simulink model "ModeloLineal_ex1"  (R2025b)
settings: Solver=VariableStepAuto  StartTime=0.0  StopTime=10.0  RelTol=1e-3
undefined symbols (not defined in the file): A, Gain, Gain2
settings Model: Creator=NMB  LastModifiedBy=NMB

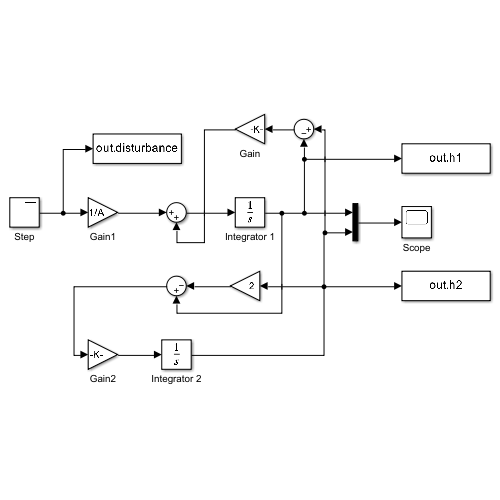
[thumbnail: Simulink's stored preview of the top-level diagram]
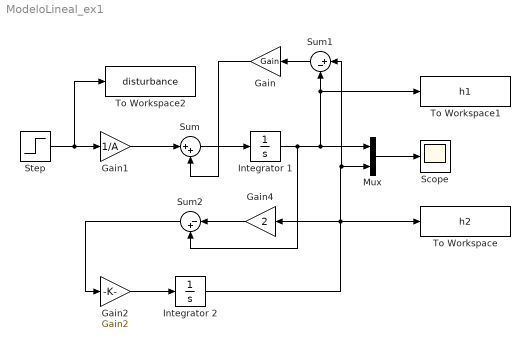
== system ModeloLineal_ex1 ==
  Gain : Gain  Gain=Gain
  Gain1 : Gain  Gain=1/A
  Gain2 : Gain  Gain=Gain2
  Gain4 : Gain  Gain=2
  Integrator 1 : Integrator
  Integrator 2 : Integrator
  Mux : Mux  Inputs=2
  Scope : Scope
  Step : Step  Time=0  After=0.5  SampleTime=0
  Sum : Sum  Inputs=|++
  Sum1 : Sum  Inputs=|+-
  Sum2 : Sum  Inputs=|-+
  To Workspace : ToWorkspace  VariableName=h2  SaveFormat=Timeseries  SampleTime=-1
  To Workspace1 : ToWorkspace  VariableName=h1  SaveFormat=Timeseries  SampleTime=-1
  To Workspace2 : ToWorkspace  VariableName=disturbance  SaveFormat=Timeseries  SampleTime=-1
  wires:
  Step/1 -> To Workspace2/1, Gain1/1
  Gain1/1 -> Sum/1
  Sum/1 -> Integrator 1/1
  Integrator 1/1 -> Mux/1, Sum1/2, To Workspace1/1, Sum2/2
  Sum1/1 -> Gain/1
  Gain/1 -> Sum/2
  Gain4/1 -> Sum2/1
  Sum2/1 -> Gain2/1
  Gain2/1 -> Integrator 2/1
  Integrator 2/1 -> Gain4/1, To Workspace/1, Sum1/1, Mux/2
  Mux/1 -> Scope/1
